simulink model "LC_Hipertenso"  (R2024b)
settings: Solver=ode15s  StartTime=0.0  StopTime=10.0  RelTol=1e-3
libraries: slpidlib x1
settings Model: Creator=leslie  LastModifiedBy=leslie
settings DataIOCC: ReturnWorkspaceOutputs=off  TimeSaveName=t  OutputSaveName=y
settings DebuggingCC: AlgebraicLoopMsg=none  ArtificialAlgebraicLoopMsg=none  MaxConsecutiveZCsMsg=none  OperatingPointInterfaceChecksumMismatchMsg=none

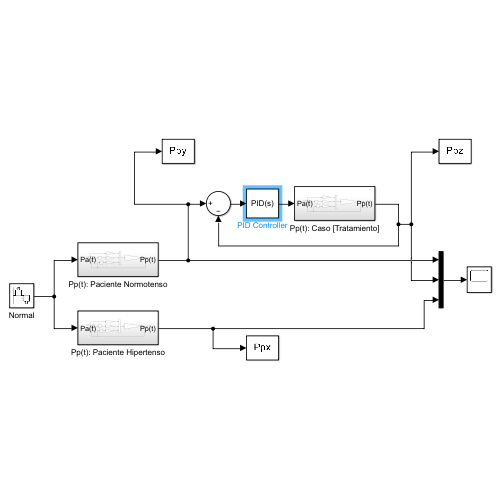
[thumbnail: Simulink's stored preview of the top-level diagram]
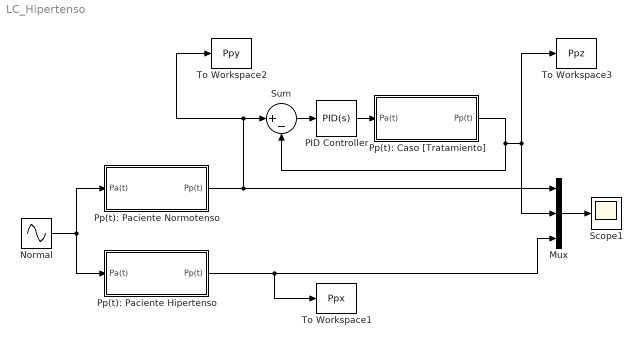
== system LC_Hipertenso ==
  Mux : Mux  Inputs=3
  Normal : Sin  Bias=0.8  Frequency=(2*pi)*(95/60)  SampleTime=0.001
  PID Controller : slpidlib/PID Controller  Controller=PID  Form=Parallel  TimeDomain=Continuous-time  UseExternalTs=off  SampleTime=-1  IntegratorMethod=Forward Euler  FilterMethod=Forward Euler  ControllerParametersSource=internal  P=0.000167674875367038  I=551.498135506255  UseKiTs=off  D=0  UseExternalDerivativeSource=off  N=100  UseFilter=on  TunerSelectOption=Transfer Function Based (PID Tuner App)  InitialConditionSource=internal  InitialConditionForIntegrator=0  InitialConditionForFilter=0  DifferentiatorICPrevScaledInput=0  ExternalReset=none  TrackingMode=off  Kt=1  LimitOutput=off  SatLimitsSource=internal  UpperSaturationLimit=inf  LowerSaturationLimit=-inf  LinearizeAsGain=on  AntiWindupMode=none  Kb=1  LimitIntegrator=off  UpperIntegratorSaturationLimit=inf  LowerIntegratorSaturationLimit=-inf  POutMin=[]  POutMax=[]  IOutMin=[]  IOutMax=[]  DOutMin=[]  DOutMax=[]  NOutMin=[]  NOutMax=[]  SumOutMin=[]  SumOutMax=[]  SaturationOutMin=[]  SaturationOutMax=[]  PParamMin=[]  PParamMax=[]  IParamMin=[]  IParamMax=[]  DParamMin=[]  DParamMax=[]  NParamMin=[]  NParamMax=[]  KbParamMin=[]  KbParamMax=[]  KtParamMin=[]  KtParamMax=[]  KbOutMin=[]  KbOutMax=[]  KtOutMin=[]  KtOutMax=[]  IntegratorOutMin=[]  IntegratorOutMax=[]  FilterOutMin=[]  FilterOutMax=[]  SumI1OutMin=[]  SumI1OutMax=[]  SumI2OutMin=[]  SumI2OutMax=[]  SumI3OutMin=[]  SumI3OutMax=[]  SumI4OutMin=[]  SumI4OutMax=[]  SumDOutMin=[]  SumDOutMax=[]  DifferentiatorOutMin=[]  DifferentiatorOutMax=[]  FilterDiffOutCoefMin=[]  FilterDiffOutCoefMax=[]  ReciprocalOutMin=[]  ReciprocalOutMax=[]  SumDenOutMin=[]  SumDenOutMax=[]  SumNumOutMin=[]  SumNumOutMax=[]  DivideOutMin=[]  DivideOutMax=[]  UdiffTsProdOutMin=[]  UdiffTsProdOutMax=[]  NTsProdOutMin=[]  NTsProdOutMax=[]  UintegralTsProdOutMin=[]  UintegralTsProdOutMax=[]  UngainTsProdOutMin=[]  UngainTsProdOutMax=[]  ClampingZeroOutDataTypeStr=Inherit: Inherit via back propagation  ClampingZeroOutMin=[]  ClampingZeroOutMax=[]  FilterDenConstantOutDataTypeStr=Inherit: Inherit via back propagation  FilterDenConstantOutMin=[]  FilterDenConstantOutMax=[]  PCopyOutDataTypeStr=Inherit: Inherit via back propagation  PCopyOutMin=[]  PCopyOutMax=[]  NCopyOutDataTypeStr=Inherit: Inherit via back propagation  NCopyOutMin=[]  NCopyOutMax=[]  IntegratorContinuousStateAttributes=''  IntegratorStateMustResolveToSignalObject=off  IntegratorRTWStateStorageClass=Auto  FilterContinuousStateAttributes=''  FilterStateMustResolveToSignalObject=off  FilterRTWStateStorageClass=Auto  ParallelPVariant=InternalParameters  IdealPVariant=Disabled  IVariant=InternalParameters  DVariant=InternalParameters  IntegratorVariant=Continuous  SatVariant=Disabled  AWVariant=Passthrough  PCopyVariant=Disabled  TRVariant=Disabled  FdbkBlocksVariant=Forward  IdealPFdbkVariant=Disabled  SatFdbkVariant=Disabled  DerivativeFilterVariant=ContFilter  NVariant=InternalParameters  NCopyVariant=Disabled  FilterICVariant=InternalICsFilter  IntegratorICVariant=InternalICs  ExternalResetVariant=Disabled  TRSumVariant=Passthrough  SumFdbkVariant=Disabled  SumVariant=Sum_PID  TsampFilterVariant=InternalTs  TsampNgainVariant=Passthrough  TsampIntegralVariant=Disabled_SignalSpec  ExternalSaturationOutDataTypeStr=Inherit: Same as second input  DerivativeSourceVariant=ErrorSignal  PreIntVariant=InternalPreInt
  Pp(t): Caso [Tratamiento] : Subsystem
  Pp(t): Paciente Hipertenso : Subsystem
  Pp(t): Paciente Normotenso : Subsystem
  Scope1 : Scope
  Sum : Sum  Inputs=|+-
  To Workspace1 : ToWorkspace  VariableName=Ppx  SaveFormat=Timeseries  SampleTime=-1
  To Workspace2 : ToWorkspace  VariableName=Ppy  SaveFormat=Timeseries  SampleTime=-1
  To Workspace3 : ToWorkspace  VariableName=Ppz  SaveFormat=Timeseries  SampleTime=-1
  wires:
  Mux/1 -> Scope1/1
  Pp(t): Paciente Hipertenso/1(Pp(t)) -> Mux/3, To Workspace1/1
  Pp(t): Paciente Normotenso/1(Pp(t)) -> To Workspace2/1, Sum/1, Mux/1
  Sum/1 -> PID Controller/1
  Normal/1 -> Pp(t): Paciente Hipertenso/1(Pa(t)), Pp(t): Paciente Normotenso/1(Pa(t))
  Pp(t): Caso [Tratamiento]/1(Pp(t)) -> Sum/2, To Workspace3/1, Mux/2
  PID Controller/1 -> Pp(t): Caso [Tratamiento]/1(Pa(t))

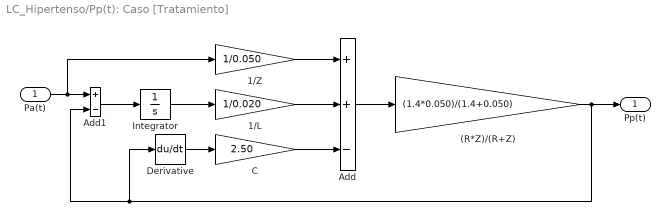
== system LC_Hipertenso/Pp(t): Caso [Tratamiento] ==
  Pa(t) : Inport
  (R*Z)/(R+Z) : Gain  Gain=(1.4*0.050)/(1.4+0.050)
  1/L : Gain  Gain=1/0.020
  1/Z : Gain  Gain=1/0.050
  Add : Sum  Inputs=++-
  Add1 : Sum  Inputs=+-
  C : Gain  Gain=2.50
  Derivative : Derivative
  Integrator : Integrator
  Pp(t) : Outport
  wires:
  Add/1 -> (R*Z)/(R+Z)/1
  Derivative/1 -> C/1
  1/Z/1 -> Add/1
  C/1 -> Add/3
  1/L/1 -> Add/2
  Integrator/1 -> 1/L/1
  Pa(t)/1 -> 1/Z/1, Add1/1
  (R*Z)/(R+Z)/1 -> Pp(t)/1, Derivative/1, Add1/2
  Add1/1 -> Integrator/1

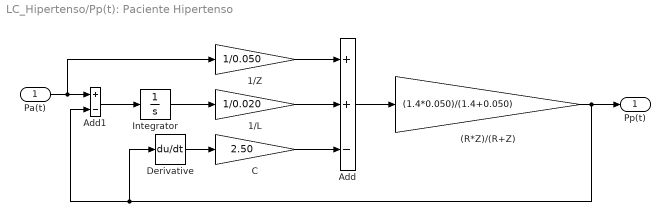
== system LC_Hipertenso/Pp(t): Paciente Hipertenso ==
  Pa(t) : Inport
  (R*Z)/(R+Z) : Gain  Gain=(1.4*0.050)/(1.4+0.050)
  1/L : Gain  Gain=1/0.020
  1/Z : Gain  Gain=1/0.050
  Add : Sum  Inputs=++-
  Add1 : Sum  Inputs=+-
  C : Gain  Gain=2.50
  Derivative : Derivative
  Integrator : Integrator
  Pp(t) : Outport
  wires:
  Add/1 -> (R*Z)/(R+Z)/1
  Derivative/1 -> C/1
  1/Z/1 -> Add/1
  C/1 -> Add/3
  1/L/1 -> Add/2
  Integrator/1 -> 1/L/1
  Pa(t)/1 -> 1/Z/1, Add1/1
  (R*Z)/(R+Z)/1 -> Pp(t)/1, Derivative/1, Add1/2
  Add1/1 -> Integrator/1

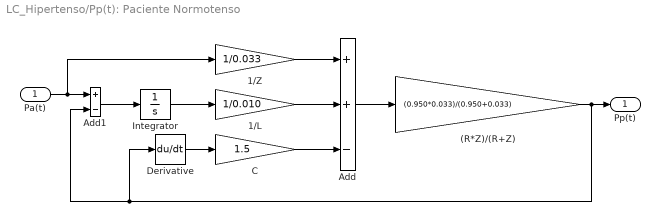
== system LC_Hipertenso/Pp(t): Paciente Normotenso ==
  Pa(t) : Inport
  (R*Z)/(R+Z) : Gain  Gain=(0.950*0.033)/(0.950+0.033)
  1/L : Gain  Gain=1/0.010
  1/Z : Gain  Gain=1/0.033
  Add : Sum  Inputs=++-
  Add1 : Sum  Inputs=+-
  C : Gain  Gain=1.5
  Derivative : Derivative
  Integrator : Integrator
  Pp(t) : Outport
  wires:
  Add/1 -> (R*Z)/(R+Z)/1
  Derivative/1 -> C/1
  1/Z/1 -> Add/1
  C/1 -> Add/3
  1/L/1 -> Add/2
  Integrator/1 -> 1/L/1
  Pa(t)/1 -> 1/Z/1, Add1/1
  (R*Z)/(R+Z)/1 -> Pp(t)/1, Derivative/1, Add1/2
  Add1/1 -> Integrator/1
